simulink model "autonomy1_first_run_Ryan"  (R2018a)
settings: Solver=VariableStepAuto  StartTime=0.0  StopTime=inf  RelTol=1e-3
InitFcn:
  | run('initArena.m')
values from neighbouring files (symbols this model uses):
  allObstacles = [1 2 3 4 5 6 7 8 9 10 11 12 ... (3348 elements, 186x3x6)]    [a.mat]    (also in initArena.m = vertcat(limit, obstacle1, obstacle2, obstacle3, obstacle4, o)
  endPt = [53 28]    [a.mat]    (also in initArena.m = horzcat(endPtx, endPty))
settings Model: Creator=alex  LastModifiedBy=Ryan Cerrone

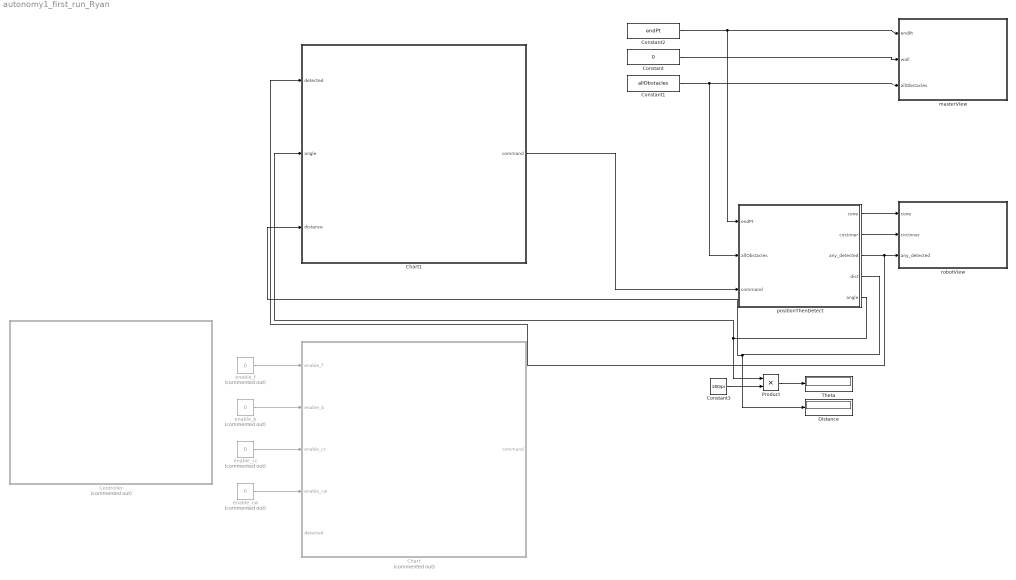
== system autonomy1_first_run_Ryan ==
  Chart : Stateflow chart  Commented=on  TreatAsAtomicUnit=on
  Chart1 : Stateflow chart  TreatAsAtomicUnit=on
  Constant : Constant  Value=0
  Constant1 : Constant  Value=allObstacles
  Constant2 : Constant  Value=endPt
  Constant3 : Constant  Value=180/pi
  Controller : Subsystem  Commented=on
  "Distance " : Display
  Product : Product
  Theta : Display
  "enable_b " : Constant  Commented=on  Value=0
  "enable_cc " : Constant  Commented=on  Value=0
  "enable_cw " : Constant  Commented=on  Value=0
  "enable_f " : Constant  Commented=on  Value=0
  masterView : MATLAB Function  TreatAsAtomicUnit=on
  positionThenDetect : MATLAB Function  TreatAsAtomicUnit=on
  robotView : MATLAB Function  TreatAsAtomicUnit=on
  wires:
  "enable_f "/1 -> Chart/1(enable_f)
  "enable_b "/1 -> Chart/2(enable_b)
  "enable_cc "/1 -> Chart/3(enable_cc)
  "enable_cw "/1 -> Chart/4(enable_cw)
  Constant/1 -> masterView/2(wall)
  Constant1/1 -> positionThenDetect/2(allObstacles), masterView/3(allObstacles)
  Chart1/1(command) -> positionThenDetect/3(command)
  positionThenDetect/1(cone) -> robotView/1(cone)
  positionThenDetect/3(any_detected) -> Chart1/1(detected), robotView/3(any_detected)
  positionThenDetect/2(circInner) -> robotView/2(circInner)
  Constant2/1 -> positionThenDetect/1(endPt), masterView/1(endPt)
  Constant3/1 -> Product/2
  positionThenDetect/5(angle) -> Chart1/2(angle), Product/1
  Product/1 -> Theta/1
  positionThenDetect/4(dist) -> Chart1/3(distance), "Distance "/1

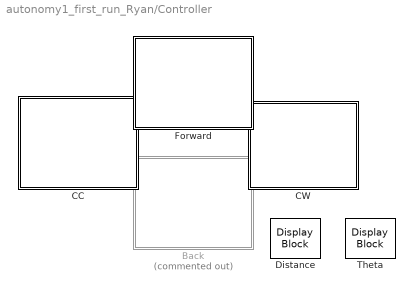
== system autonomy1_first_run_Ryan/Controller ==
  Back : Subsystem  Commented=on  DialogController=hmiCreateDDGDialog  IsWebBlock=on  mask(MWDashboardBlock){webBlockId=1a5e94ef-030e-49cd-b944-b929b04abc70, webBlockType=pushbutton, ShowInLibBrwoser=on, ShowInitialText=on, HMISrcModelName=autonomy1_first_run_Ryan}
      mask prompts: webBlockId "WebBlock Id"; webBlockType "WebBlock Type"; HMISrcModelName "Source Model"
      mask help: SimulinkHMI:dialogs:PushButtonDialogDesc
      mask Help: helpview([docroot '/mapfiles/simulink.map'], 'hmi_push_button')
      mask Display:
      | model = bdroot(gcb);
      | if strcmp(get_param(model,'BlockDiagramType'), 'library')
      |     image([(matlabroot) '/toolbox/simulink/hmi/icons/PushButton.png']);
      | end
  "CC " : Subsystem  DialogController=hmiCreateDDGDialog  IsWebBlock=on  mask(MWDashboardBlock){webBlockId=f6d6ee6b-2047-45ee-ab2e-570b521bf019, webBlockType=pushbutton, ShowInLibBrwoser=on, ShowInitialText=on, HMISrcModelName=autonomy1_first_run_Ryan}
      mask prompts: webBlockId "WebBlock Id"; webBlockType "WebBlock Type"; HMISrcModelName "Source Model"
      mask help: SimulinkHMI:dialogs:PushButtonDialogDesc
      mask Help: helpview([docroot '/mapfiles/simulink.map'], 'hmi_push_button')
      mask Display:
      | model = bdroot(gcb);
      | if strcmp(get_param(model,'BlockDiagramType'), 'library')
      |     image([(matlabroot) '/toolbox/simulink/hmi/icons/PushButton.png']);
      | end
  "CW " : Subsystem  DialogController=hmiCreateDDGDialog  IsWebBlock=on  mask(MWDashboardBlock){webBlockId=5b3cd59d-fae2-469c-adcb-5a1af564bf62, webBlockType=pushbutton, ShowInLibBrwoser=on, ShowInitialText=on, HMISrcModelName=autonomy1_first_run_Ryan}
      mask prompts: webBlockId "WebBlock Id"; webBlockType "WebBlock Type"; HMISrcModelName "Source Model"
      mask help: SimulinkHMI:dialogs:PushButtonDialogDesc
      mask Help: helpview([docroot '/mapfiles/simulink.map'], 'hmi_push_button')
      mask Display:
      | model = bdroot(gcb);
      | if strcmp(get_param(model,'BlockDiagramType'), 'library')
      |     image([(matlabroot) '/toolbox/simulink/hmi/icons/PushButton.png']);
      | end
  Distance : DisplayBlock  WebBlockId=66  LabelPosition=Hide
  Forward : Subsystem  DialogController=hmiCreateDDGDialog  IsWebBlock=on  mask(MWDashboardBlock){webBlockId=418d2ee9-92ed-471b-995b-1589f387356b, webBlockType=pushbutton, ShowInLibBrwoser=on, ShowInitialText=on, HMISrcModelName=autonomy1_first_run_Ryan}
      mask prompts: webBlockId "WebBlock Id"; webBlockType "WebBlock Type"; HMISrcModelName "Source Model"
      mask help: SimulinkHMI:dialogs:PushButtonDialogDesc
      mask Help: helpview([docroot '/mapfiles/simulink.map'], 'hmi_push_button')
      mask Display:
      | model = bdroot(gcb);
      | if strcmp(get_param(model,'BlockDiagramType'), 'library')
      |     image([(matlabroot) '/toolbox/simulink/hmi/icons/PushButton.png']);
      | end
  Theta : DisplayBlock  WebBlockId=67  LabelPosition=Hide

== system autonomy1_first_run_Ryan/Controller/Back ==

== system autonomy1_first_run_Ryan/Controller/CC  ==

== system autonomy1_first_run_Ryan/Controller/CW  ==

== system autonomy1_first_run_Ryan/Controller/Forward ==

== stateflow chart autonomy1_first_run_Ryan/Chart1 ==
  settings: stateMachineType=MOORE_MACHINE
  state no_input
    command = 5
  state point_to_dot_ccw
    command = 5
  state point_to_dot_cw
    command = 5
  state forward
    command = 1
  state stop1
    command = 0
  state rotate_away
    command = 3
  state forward1
    command = 1
  state stop
    command = 0
  state rotate_to_dot_again_cc
    command = 3
  state rotate_to_dot_again_cw
    command = 4
  state rotate_away1
    command = 3
  (default) -> no_input
  no_input -> point_to_dot_ccw [order 1] : [ angle < -pi/128]
  point_to_dot_ccw -> no_input
  no_input -> forward [order 2] : [angle > -pi/128 & angle < pi/128]
  no_input -> point_to_dot_cw [order 3] : [angle > pi/128]
  point_to_dot_cw -> no_input
  forward -> stop1 [order 3] : [distance < 250]
  forward -> forward1 [order 1] : [angle > pi/128 | angle < -pi/128]
  forward -> rotate_away [order 2] : [detected == 1]
  rotate_away -> forward : [detected == 0]
  rotate_to_dot_again_cw -> forward1 : [angle > -pi/128 & angle < pi/128 | detected == 0]
  rotate_to_dot_again_cc -> forward1 : [angle > -pi/128 & angle < pi/128 | detected == 0]
  forward1 -> rotate_to_dot_again_cc [order 4] : [detected == 1 & angle < -pi/128 ]
  forward1 -> rotate_to_dot_again_cw [order 1] : [detected == 1 & angle > pi/128]
  rotate_away1 -> forward1 : [detected == 0]
  forward1 -> rotate_away1 [order 3] : [detected == 1 & distance > 700]
  forward1 -> stop [order 2] : [distance < 250]
  data: command output; detected input; angle input; distance input

== matlab function autonomy1_first_run_Ryan/positionThenDetect ==
  data: endPt input; allObstacles input; cone output; command input; circInner output; any_detected output; dist output; angle output
function [cone, circInner, any_detected, dist, angle] = positionThenDetect(endPt, allObstacles, command) % put in starting position
                                                                                                         %call astar ONCE in the beginning
                                                                                                         %make robot follow path from there
    persistent xpos ypos theta
    
    % Define start location
    if isempty(xpos)
        xpos = randi([10,50]);
        ypos = randi([2,5]);
        theta = pi/4;
    end
    % Initaize stored values for discovered objects 
    
    % Robot specifications   
    botRadius = 2;
    coneDepth = 3;
    speed = 10;
    turnSpeed = pi/128;

    % Radius of robot vision and representing circles 
    r = sqrt(botRadius^2+(2*coneDepth^2)-2*botRadius*sqrt(2*coneDepth^2)*cos(135*pi/180));
    t = linspace(-pi,pi);
    xc = [r*cos(t); botRadius*cos(t)];
    yc = [-r*sin(t); -botRadius*sin(t)];

    % Update position and rotation based on command 
    if command == 1 % forward
        xpos = xpos + speed*cos(theta);
        ypos = ypos + speed*sin(theta);
    elseif command == 2 % back
        xpos = xpos - speed*cos(theta);
        ypos = ypos - speed*sin(theta);
    elseif command == 3 % counter clockwise
        theta = theta + turnSpeed;
    elseif command == 4 % clockwise 
        theta = theta - turnSpeed;
    end
    if theta >= 2*pi
        theta = theta - 2*pi;
    elseif theta <= -2*pi
        theta = theta + 2*pi;
    end

    % Calculate rotated cone around origin 
    thigh = theta + asin(coneDepth/r);
    tlow = thigh-2*asin(coneDepth/r);
    x = [botRadius*cos(theta) r*cos(thigh) r*cos(tlow) botRadius*cos(theta)];
    y = [botRadius*sin(theta) r*sin(thigh) r*sin(tlow) botRadius*sin(theta)];
    z = zeros(1,4);
    rotated_cone = fliplr(rot90(vertcat(x,y,z),3));
        
    % Translate cone to new position 
    cone = rotated_cone;
    cone(:,1) = rotated_cone(:,1) + xpos;
    cone(:,2) = rotated_cone(:,2) + ypos;
    cone(:,3) = rotated_cone(:,3);
    
    % Translate circle to new position 
    circInner = zeros(2, length(t));
    circInner(1,:) = xc(2,:) + xpos;
    circInner(2,:) = yc(2,:) + ypos;

    % Check if obstacle is in vision cone 
    detected = detectRotated(allObstacles, cone);
    
    % Update stored values of discovered objects  
    
    % Indicate if any obstacles are detected 
    any_detected = double(any(detected(:)));
    
    % Calculate intantaneous angle/dist between current and ideal orientation 
    angle = degFromPath(endPt, xpos, ypos, theta); 
    dist = distFromPath(endPt, xpos, ypos);
   
end

== stateflow chart autonomy1_first_run_Ryan/Chart ==
  settings: stateMachineType=MOORE_MACHINE
  state no_input
    command = 0
  state check_detected
  state back
    command = 2
  state counter_clockwise
    command = 3
  state clockwise
    command = 4
  state forward
    command = 1
  (default) -> no_input
  no_input -> check_detected [order 1] : [enable_f == 1]
  forward -> no_input [order 1] : [enable_f == 0]
  check_detected -> no_input [order 2] : [detected==1]
  no_input -> back [order 4] : [enable_b ==1]
  back -> no_input : [enable_b== 0]
  no_input -> counter_clockwise [order 3] : [enable_cc == 1]
  counter_clockwise -> no_input : [enable_cc == 0]
  no_input -> clockwise [order 2] : [enable_cw == 1]
  clockwise -> no_input : [enable_cw == 0]
  forward -> check_detected [order 2] : [detected==1]
  check_detected -> forward [order 1] : [detected==0]
  data: enable_f input; enable_b input; enable_cc input; enable_cw input; command output; detected input

== matlab function autonomy1_first_run_Ryan/masterView ==
  data: endPt input; wall input; allObstacles input
function masterView(endPt, wall, allObstacles)
    % Visualize data
    %plot(wall(:,1), wall(:,2), 'ks-');
    hold on 
    grid on
    grid minor
    xlim([0 5756]);
    ylim([0 3691]);
    xlabel('Field Width (mm)')
    ylabel('Field Height (mm)')
    title('2D Mining Robot Simulation')
    plot(allObstacles(:,1), allObstacles(:,2), 'b.');
    plot(endPt(1), endPt(2), 'g*');
end

== matlab function autonomy1_first_run_Ryan/robotView ==
  data: cone input; circInner input; any_detected input
function robotView(cone, circInner, any_detected)
    if any_detected
        coneColor = 'r';
    else
        coneColor = 'k';
    end
    
    coneFig = plot(cone(:,1),cone(:,2), coneColor);
    circOFig = plot(circInner(1,:),circInner(2,:));
    set([coneFig circOFig],'LineWidth', 5)
    hold off
end
